simulink model "j123"  (R2021b)
settings: Solver=VariableStepAuto  StartTime=0.0  StopTime=1e-4  RelTol=1e-3
libraries: dsparch4 x1
settings Model: Creator=zhonghuatu  LastModifiedBy=zhonghuatu
settings DataIOCC: ExternalInput=[ts,urs]

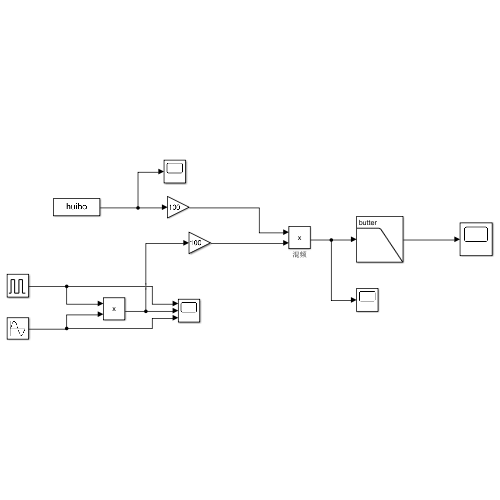
[thumbnail: Simulink's stored preview of the top-level diagram]
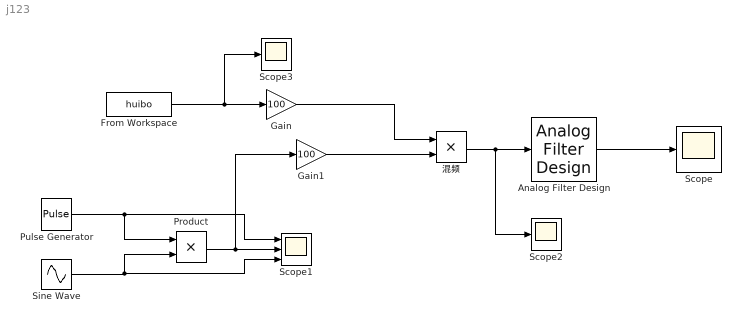
== system j123 ==
  Analog Filter Design : dsparch4/Analog Filter Design  method=Butterworth  filttype=Lowpass  N=8  Wlo=2.1e3  Whi=80  Rp=2  Rs=40
  From Workspace : FromWorkspace  VariableName=huibo  SampleTime=-1
  Gain : Gain  Gain=100
  Gain1 : Gain  Gain=100
  Product : Product
  Pulse Generator : DiscretePulseGenerator  PulseType=Time based  Period=20e-6  PulseWidth=50  VectorParams1D=off
  Scope : Scope
  Scope1 : Scope  NumInputPorts=3
  Scope2 : Scope
  Scope3 : Scope
  Sine Wave : Sin  Amplitude=100  Frequency=100e6*2*pi  Phase=10*pi/180  SampleTime=0
  混频 : Product
  wires:
  混频/1 -> Scope2/1, Analog Filter Design/1
  Pulse Generator/1 -> Scope1/1, Product/1
  Sine Wave/1 -> Scope1/3, Product/2
  Product/1 -> Gain1/1, Scope1/2
  From Workspace/1 -> Scope3/1, Gain/1
  Gain/1 -> 混频/1
  Gain1/1 -> 混频/2
  Analog Filter Design/1 -> Scope/1
